simulink model "PWM2"  (Simulink 10.0)
settings: Solver=ode1  StartTime=0.0  StopTime=inf  FixedStep=0.01  MaxStep=0.02  RelTol=1e-3  AbsTol=1e-6
settings Model: Creator=Admin  LastModifiedBy=bhisma  SimulationMode=external  ExtModeTrigDuration=10000
settings ConfigSet: Description=rtmc9s12target_R2009b
settings SolverCC: AutoScaleAbsTol=off
settings DataIOCC: SignalLoggingSaveFormat=ModelDataLogs  SaveOutput=off  SaveTime=off  SignalLoggingName=sigsOut
settings OptimizationCC: BlockReduction=off  BooleanDataType=off  ExpressionDepthLimit=2147483647  InitFltsAndDblsToZero=on  LifeSpan=1  EfficientTunableParamExpr=on
settings DebuggingCC: SaveWithParameterizedLinksMsg=none  SignalResolutionControl=TryResolveAllWithWarning  MultiTaskDSMMsg=warning  MultiTaskCondExecSysMsg=none  FcnCallInpInsideContextMsg=warning  StateNameClashWarn=warning
settings HardwareCC: ProdBitPerInt=16  ProdBitPerPointer=16  ProdBitPerSizeT=16  ProdBitPerPtrDiffT=16  ProdEndianess=BigEndian  ProdWordSize=16  ProdHWDeviceType=Motorola HC12
settings SFSimCC: MATLABDynamicMemAlloc=off
settings RTWCC: SystemTargetFile=mc9s12.tlc  GenerateMakefile=off  TemplateMakefile=mc9s12.tmf
settings CodeAppCC: IgnoreCustomStorageClasses=off  CustomSymbolStrType=$N$R$M  InternalIdentifier=Classic
settings STFCustomTargetCC: TargetFcnLib=ansi_tfl_tmw.mat  ModelReferenceCompliant=off  IncludeMdlTerminateFcn=off  ERTCustomFileBanners=on  SupportNonInlinedSFcns=off  RemoveResetFunc=on  MATLABClassNameForMDSCustomization=Simulink.SoftwareTarget.ERTCustomization  CPPClassGenCompliant=on  SystemTargetFile=mc9s12.tlc
settings ERTTargetCC: TargetFcnLib=ansi_tfl_tmw.mat  MultiwordLength=2048  ModelReferenceCompliant=off  ParMdlRefBuildCompliant=off  CompOptLevelCompliant=off  ConcurrentExecutionCompliant=off  IncludeMdlTerminateFcn=off  CombineOutputUpdateFcns=off  SupportContinuousTime=on  ModelStepFunctionPrototypeControlCompliant=off  GRTInterface=on  UseToolchainInfoCompliant=off  ExtMode=on  ExtModeMexFile=ext_serial_mc9s12_comm  ExtModeMexArgs=1,2,115200  ERTCustomFileTemplate=mc9s12_file_process.tlc  ConvertIfToSwitch=off  SuppressUnreachableDefaultCases=off
settings CustomProperty: DataType=RTWOptions_EnumType_C__Users_fw__SVN_rtmc9s12-target_trunk_rtmc9s12_CW_R2009b_bin_mc9s12_1mc9s12_TargetBoard  Value=Dragon12Plus
settings EnumStrPairs: String=Dragon12
settings ConfigComp: CovExternalEMLEnable=off

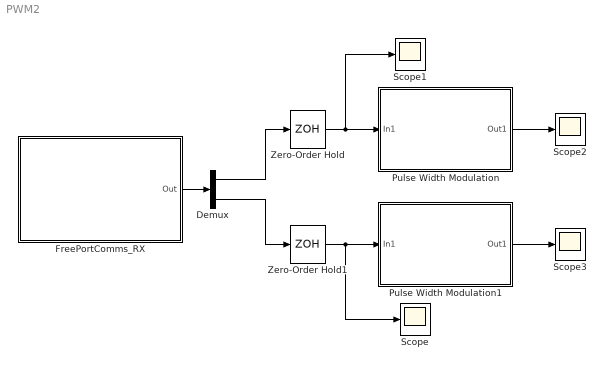
== system PWM2 ==
  Demux : Demux  Outputs=2
  FreePortComms_RX : Subsystem  Tag=mcTarget_freePortCommsRX  mask{sampletime=0.1, port=SCI0, baudrate=115200, channel=0, buf_size=2, data_type=SINGLE, format=off, outformat=on}
      mask prompts: sampletime "Sample time"; port "Communication port"; channel "Channel number"; buf_size "Number of elements"; data_type "Data Type"; format "Block receives raw data"; outformat "Block output is double"
      mask init:
      | [buf_sizestr, portNamestr, baudratestr, channelstr, data_type_str, sampletime_str] = mbc_freeportrxd(sampletime, port, baudrate, channel, buf_size, data_type, format, outformat);
      mask Help: web('freePortComms_rxd.html');
      mask TypeOptions port: SCI0 | SCI1 | COM1 | COM2 | COM3 | COM4
      mask TypeOptions baudrate: 300 | 600 | 1200 | 2400 | 4800 | 9600 | 19200 | 38400 | 57600 | 115200
      mask TypeOptions data_type: SINGLE | INT8 | UINT8 | INT16 | UINT16 | INT32 | UINT32 | BOOLEAN
      mask Display: fprintf('Receive %s element(s)\nComm port: %s\nBaudrate: %s bps\nChannel: %s\nData type: %s\n Sample rate: %s', buf_sizestr, portNamestr, baudratestr, channelstr, data_type_str, sampletime_str)
  Pulse Width Modulation : Subsystem  Tag=mcTarget_pwm  mask{sampletime=0.01, resolution=16 bit, PWMperiod=0.5, pulse_pin=1  (8-bit / 16-bit), sign_port=PTH, sign_pin=1, Vmax=5, sig_mon=on}
      mask prompts: sampletime "Sample time"; PWMperiod "PWM period (8-bit : up to 0.699 s, 16-bit : up to 179 s)"; pulse_pin "Pulse pin (PTP)"; sign_port "Sign port"; sign_pin "Sign pin"; Vmax "Saturation input level [simulated voltage]"; sig_mon "Signal monitoring"
      mask init:
      | [pulsepinstr, signportstr, signpinstr, periodstr, clkABstr, resstr] = mbc_pwmoutput(sampletime, resolution, PWMperiod, pulse_pin, sign_port, sign_pin, Vmax, sig_mon);
      mask Help: web('pwm_sfcn_9S12.html');
      mask TypeOptions resolution: 8 bit | 16 bit
      mask TypeOptions pulse_pin: 0  (8-bit) | 1  (8-bit / 16-bit) | 2  (8-bit) | 3  (8-bit / 16-bit) | 4  (8-bit) | 5  (8-bit / 16-bit) | 6  (8-bit) | 7  (8-bit / 16-bit)
      mask TypeOptions sign_port: PORTA | PORTB | PTH | PTJ | PTM | PTP | PTT | PTS
      mask TypeOptions sign_pin: 0 | 1 | 2 | 3 | 4 | 5 | 6 | 7
      mask Display: fprintf('PWM-%s, %s-bit\nPulse pin: PTP.%s\nSign pin: %s.%s\nPeriod: %s (s)\nSaturation: %d', clkABstr, resstr, pulsepinstr, signportstr, signpinstr, periodstr, Vmax)
  Pulse Width Modulation1 : Subsystem  Tag=mcTarget_pwm  mask{sampletime=0.01, resolution=16 bit, PWMperiod=0.5, pulse_pin=3  (8-bit / 16-bit), sign_port=PTH, sign_pin=2, Vmax=5, sig_mon=on}
      mask prompts: sampletime "Sample time"; PWMperiod "PWM period (8-bit : up to 0.699 s, 16-bit : up to 179 s)"; pulse_pin "Pulse pin (PTP)"; sign_port "Sign port"; sign_pin "Sign pin"; Vmax "Saturation input level [simulated voltage]"; sig_mon "Signal monitoring"
      mask init:
      | [pulsepinstr, signportstr, signpinstr, periodstr, clkABstr, resstr] = mbc_pwmoutput(sampletime, resolution, PWMperiod, pulse_pin, sign_port, sign_pin, Vmax, sig_mon);
      mask Help: web('pwm_sfcn_9S12.html');
      mask TypeOptions resolution: 8 bit | 16 bit
      mask TypeOptions pulse_pin: 0  (8-bit) | 1  (8-bit / 16-bit) | 2  (8-bit) | 3  (8-bit / 16-bit) | 4  (8-bit) | 5  (8-bit / 16-bit) | 6  (8-bit) | 7  (8-bit / 16-bit)
      mask TypeOptions sign_port: PORTA | PORTB | PTH | PTJ | PTM | PTP | PTT | PTS
      mask TypeOptions sign_pin: 0 | 1 | 2 | 3 | 4 | 5 | 6 | 7
      mask Display: fprintf('PWM-%s, %s-bit\nPulse pin: PTP.%s\nSign pin: %s.%s\nPeriod: %s (s)\nSaturation: %d', clkABstr, resstr, pulsepinstr, signportstr, signpinstr, periodstr, Vmax)
  Scope{,1..3} (4 alike) : Scope
  Zero-Order Hold : ZeroOrderHold  SampleTime=0.01
  Zero-Order Hold1 : ZeroOrderHold  SampleTime=0.01
  wires:
  Zero-Order Hold/1 -> Scope1/1, Pulse Width Modulation/1(In1)
  Zero-Order Hold1/1 -> Scope/1, Pulse Width Modulation1/1(In1)
  FreePortComms_RX/1(Out) -> Demux/1
  Demux/1 -> Zero-Order Hold/1
  Demux/2 -> Zero-Order Hold1/1
  Pulse Width Modulation1/1(Out1) -> Scope3/1
  Pulse Width Modulation/1(Out1) -> Scope2/1

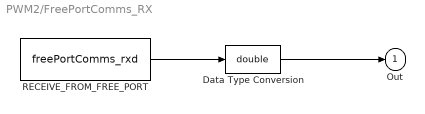
== system PWM2/FreePortComms_RX ==
  Data Type Conversion : DataTypeConversion  OutDataTypeStr=double  SaturateOnIntegerOverflow=on  RndMeth=Zero
  RECEIVE_FROM_FREE_PORT : S-Function  Tag=mcTarget_freePortCommsRX  FunctionName=freePortComms_rxd  Parameters=sampletime, channel, buf_size, data_type, port, baudrate, format  SFunctionDeploymentMode=off  EnableBusSupport=off
  Out : Outport
  wires:
  RECEIVE_FROM_FREE_PORT/1 -> Data Type Conversion/1
  Data Type Conversion/1 -> Out/1

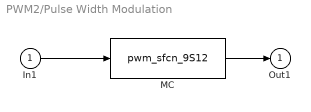
== system PWM2/Pulse Width Modulation ==
  In1 : Inport
  MC : S-Function  Tag=mcTarget_pwm  FunctionName=pwm_sfcn_9S12  Parameters=sampletime, PWMperiod, pulse_pin, sign_port, sign_pin, Vmax, sig_mon  SFunctionDeploymentMode=off  EnableBusSupport=off
  Out1 : Outport
  wires:
  In1/1 -> MC/1
  MC/1 -> Out1/1

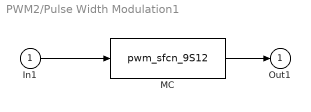
== system PWM2/Pulse Width Modulation1 ==
  In1 : Inport
  MC : S-Function  Tag=mcTarget_pwm  FunctionName=pwm_sfcn_9S12  Parameters=sampletime, PWMperiod, pulse_pin, sign_port, sign_pin, Vmax, sig_mon  SFunctionDeploymentMode=off  EnableBusSupport=off
  Out1 : Outport
  wires:
  MC/1 -> Out1/1
  In1/1 -> MC/1
